simulink model "FIR_FILTER"  (R2020b)
settings: Solver=VariableStepAuto  StartTime=0.0  StopTime=10  RelTol=1e-3
settings Model: Creator=hp  LastModifiedBy=hp
settings DataIOCC: SaveOutput=off  SaveTime=off

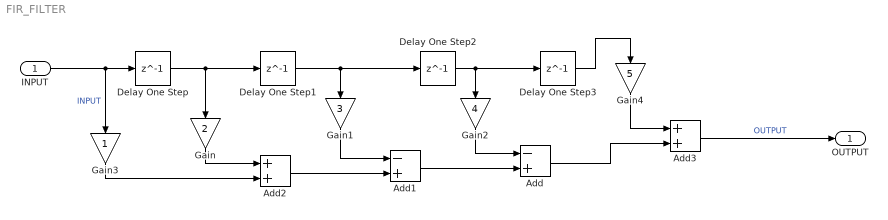
== system FIR_FILTER ==
  INPUT : Inport  OutDataTypeStr=double  PortDimensions=1  SampleTime=0
  Add : Sum  Inputs=-+
  Add1 : Sum  Inputs=-+
  Add2 : Sum
  Add3 : Sum
  Delay One Step{,1..3} (4 alike) : Delay  DelayLength=1
  Gain : Gain  Gain=2
  Gain1 : Gain  Gain=3
  Gain2 : Gain  Gain=4
  Gain3 : Gain
  Gain4 : Gain  Gain=5
  OUTPUT : Outport  OutDataTypeStr=double  PortDimensions=1  SampleTime=0
  wires:
  Gain4/1 -> Add3/1
  Delay One Step1/1 -> Gain1/1, Delay One Step2/1
  Delay One Step2/1 -> Delay One Step3/1, Gain2/1
  INPUT/1 -> Gain3/1, Delay One Step/1  "INPUT"
  Delay One Step3/1 -> Gain4/1
  Delay One Step/1 -> Gain/1, Delay One Step1/1
  Gain2/1 -> Add/1
  Add3/1 -> OUTPUT/1  "OUTPUT"
  Add1/1 -> Add/2
  Gain1/1 -> Add1/1
  Add2/1 -> Add1/2
  Gain/1 -> Add2/1
  Gain3/1 -> Add2/2
  Add/1 -> Add3/2
